simulink model "FOC_IM_discrete"  (R2018b)
settings: Solver=ode45  StartTime=0.0  StopTime=0.1  RelTol=1e-6
undefined symbols (not defined in the file): DiscIntNeverNeededParam, fs, In, J, Ki_d, Ki_q, Ki_speed, Kp_d, Kp_q, Kp_speed, landa_r, Lm, Lr, Ls, Omegae, p, plecs, Rr, Rs, T_rated, Ts, Udc, Un
libraries: powerlib_meascontrol x1, powerlib x1
settings Model: SimulationMode=accelerator  Creator=estef  LastModifiedBy=estef
settings DebuggingCC: MaxConsecutiveZCsMsg=warning

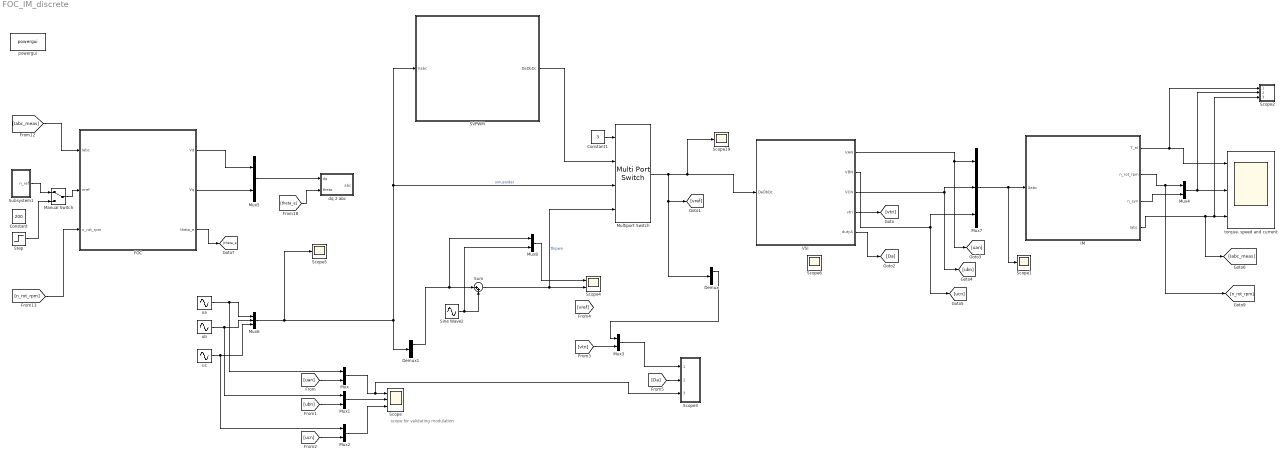
== system FOC_IM_discrete ==
  note: scope for validating modulation
  Constant : Constant  Value=200
  Constant1 : Constant  Value=3
  Demux : Demux  Outputs=3
  Demux1 : Demux  Outputs=3
  "FOC " : Subsystem
  "IM " : Subsystem
  Manual Switch : ManualSwitch
  Multiport Switch : MultiPortSwitch
  Mux{,1..5,8} (7 alike) : Mux  Inputs=2
  Mux6 : Mux  Inputs=3
  Mux7 : Mux  Inputs=3
  "SVPWM " : Subsystem
  Scope : Scope  NumInputPorts=3
  Scope{1,5..6,19} (4 alike) : Scope
  Scope2 : Subsystem  LoadFcn=plecs('sl', 300);  InitFcn=plecs('sl', 314);  StartFcn=plecs('sl', 308);  StopFcn=plecs('sl', 309);  mask{Settings=<binary blob, 1484 chars, not shown>}
      mask init:
      | plecs('sl', 315);
      settings: CopyFcn=plecs('sl', 303);  DeleteFcn=plecs('sl', 305);  UndoDeleteFcn=plecs('sl', 306);  PreSaveFcn=plecs('sl', 311);  NameChangeFcn=plecs('sl', 310);  DestroyFcn=plecs('sl', 307);  OpenFcn=plecs('sl', 302);  ErrorFcn=plerrorfcn
      mask Display: plot([0.1 0.9 0.9 0.1 0.1], [0.9 0.9 0.5 0.5 0.9])
  Scope3 : Subsystem  LoadFcn=plecs('sl', 300);  InitFcn=plecs('sl', 314);  StartFcn=plecs('sl', 308);  StopFcn=plecs('sl', 309);  mask{Settings=<binary blob, 1328 chars, not shown>}
      mask init:
      | plecs('sl', 315);
      settings: CopyFcn=plecs('sl', 303);  DeleteFcn=plecs('sl', 305);  UndoDeleteFcn=plecs('sl', 306);  PreSaveFcn=plecs('sl', 311);  NameChangeFcn=plecs('sl', 310);  DestroyFcn=plecs('sl', 307);  OpenFcn=plecs('sl', 302);  ErrorFcn=plerrorfcn
      mask Display: plot([0.1 0.9 0.9 0.1 0.1], [0.9 0.9 0.5 0.5 0.9])
  Scope4 : Scope  NumInputPorts=2
  Sine Wave2 : Sin  Amplitude=sqrt(2)*Un/5  Frequency=3*Omegae  SampleTime=0
  Step : Step  Time=0.2  After=500  SampleTime=0
  Subsystem1 : Subsystem
  Sum : Sum  Inputs=|++
  VSI : Subsystem
  dq 2 abc : Subsystem
  powergui : powerlib/powergui  Priority=1  SimulationMode=Continuous  SampleTime=50e-6  frequency=60  Iterations=50  frequencyindice=60  Pbase=100e6  ErrMax=1e-4  UnitsV=kV  UnitsW=MW  buscounter=0  FunctionMessages=off  echomessages=off  EnableUseOfTLC=off  CurrentSourceSwitches=off  DisableSnubberDevices=off  DisableRonSwitches=off  DisableVfSwitches=off  DisplayEquations=off  SolverType=Tustin/Backward Euler (TBE)  Interpol=off  ExternalGateDelay=off  methode=off  Ts=100  x0status=blocks  SPID=on  SwTol=0  HookPort=off  RestoreLinks=warning  ResistiveCurrentMeasurement=off  Frange=[0:2:500]  Ylog=off  Xlog=on  ShowGrid=off  save=off  variable=ZData  structure=phase_V  ZoomFFT=off  StartTime=0.1  cycles=10  DisplayStyle=1  fundamental=58  FreqAxis=off  MaxFrequency=1000  frequencyindicesteady=1  RmsSteady=1  display=off
  "torque, speed and current " : Scope  NumInputPorts=3
  ua : Sin  Amplitude=sqrt(2)*Un  Frequency=Omegae  SampleTime=0
  ub : Sin  Amplitude=sqrt(2)*Un  Frequency=Omegae  Phase=-2*pi/3  SampleTime=0
  uc : Sin  Amplitude=sqrt(2)*Un  Frequency=Omegae  Phase=2*pi/3  SampleTime=0
  wires:
  Mux7/1 -> Scope1/1, "IM "/1("Uabc ")
  ub/1 -> Mux1/1, Mux6/2
  [ubn] -> Mux1/2
  [ucn] -> Mux2/2
  [theta_e] -> dq 2 abc/2(theta)
  VSI/3(VCN) -> Mux7/3, [ucn]
  ua/1 -> Mux/1, Mux6/1
  [uan] -> Mux/2
  Mux1/1 -> Scope/2
  Mux5/1 -> dq 2 abc/1(dq)
  "IM "/1(T_el) -> Scope2/1(1), "torque, speed and current "/1
  uc/1 -> Mux2/1, Mux6/3
  VSI/1("VAN ") -> [uan], Mux7/1
  Mux2/1 -> Scope/3
  VSI/2("VBN ") -> Mux7/2, [ubn]
  Mux/1 -> Scope3/3(3), Scope/1
  "IM "/4(Iabc) -> [Iabc_meas], Scope2/3(3), "torque, speed and current "/3
  "FOC "/1(Vd) -> Mux5/1
  [Iabc_meas] -> "FOC "/1("Iabc ")
  "FOC "/2("Vq ") -> Mux5/2
  [n_rot_rpm] -> "FOC "/3("n_rot_rpm ")
  Manual Switch/1 -> "FOC "/2(nref)
  Subsystem1/1(n_ref) -> Manual Switch/1
  "FOC "/3("theta_e ") -> [theta_e]
  Mux4/1 -> Scope2/2(2), "torque, speed and current "/2
  "IM "/2("n_rot_rpm ") -> [n_rot_rpm], Mux4/1
  "IM "/3("n_syn ") -> Mux4/2
  Step/1 -> Manual Switch/2
  Constant1/1 -> Multiport Switch/1
  Multiport Switch/1 -> Demux/1, [vref], Scope19/1, VSI/1(DaDbDc)
  "SVPWM "/1(DaDbDc) -> Multiport Switch/2
  Mux6/1 -> Scope5/1, Multiport Switch/3, "SVPWM "/1("Vabc "), Demux1/1  "sinusoidal"
  Sine Wave2/1 -> Mux8/2, Sum/2
  Sum/1 -> Scope4/2, Multiport Switch/4  "thipwn"
  VSI/4("vtri ") -> [vtri]
  [vtri] -> Mux3/2
  Mux3/1 -> Scope3/1(1)
  VSI/5("dutyA ") -> [Da]
  [Da] -> Scope3/2(2)
  Demux/1 -> Mux3/1
  Demux1/1 -> Mux8/1, Sum/1
  Mux8/1 -> Scope4/1

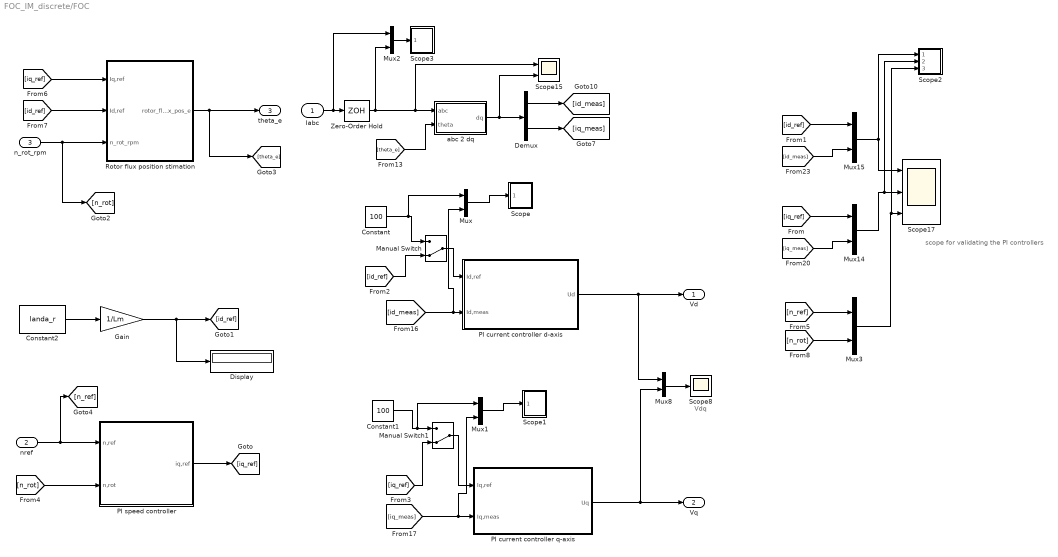
== system FOC_IM_discrete/FOC  ==
  note: scope for validating the PI controllers
  note: Vdq
  "Iabc " : Inport
  nref : Inport  Port=2
  "n_rot_rpm " : Inport  Port=3
  Constant : Constant  Value=100
  Constant1 : Constant  Value=100
  Constant2 : Constant  Value=landa_r
  Demux : Demux  Outputs=2
  Display : Display
  Gain : Gain  Gain=1/Lm
  Manual Switch : ManualSwitch  CurrentSetting=0
  Manual Switch1 : ManualSwitch  CurrentSetting=0
  Mux{,1..3,8,14..15} (7 alike) : Mux  Inputs=2
  PI current controller d-axis : Subsystem
  PI current controller q-axis : Subsystem
  PI speed controller : Subsystem
  Rotor flux position stimation : Subsystem
  Scope : Subsystem  LoadFcn=plecs('sl', 300);  InitFcn=plecs('sl', 314);  StartFcn=plecs('sl', 308);  StopFcn=plecs('sl', 309);  mask{Settings=<binary blob, 1052 chars, not shown>}
      mask init:
      | plecs('sl', 315);
      settings: CopyFcn=plecs('sl', 303);  DeleteFcn=plecs('sl', 305);  UndoDeleteFcn=plecs('sl', 306);  PreSaveFcn=plecs('sl', 311);  NameChangeFcn=plecs('sl', 310);  DestroyFcn=plecs('sl', 307);  OpenFcn=plecs('sl', 302);  ErrorFcn=plerrorfcn
      mask Display: plot([0.1 0.9 0.9 0.1 0.1], [0.9 0.9 0.5 0.5 0.9])
  Scope1 : Subsystem  LoadFcn=plecs('sl', 300);  InitFcn=plecs('sl', 314);  StartFcn=plecs('sl', 308);  StopFcn=plecs('sl', 309);  mask{Settings=<binary blob, 1052 chars, not shown>}
      mask init:
      | plecs('sl', 315);
      settings: CopyFcn=plecs('sl', 303);  DeleteFcn=plecs('sl', 305);  UndoDeleteFcn=plecs('sl', 306);  PreSaveFcn=plecs('sl', 311);  NameChangeFcn=plecs('sl', 310);  DestroyFcn=plecs('sl', 307);  OpenFcn=plecs('sl', 302);  ErrorFcn=plerrorfcn
      mask Display: plot([0.1 0.9 0.9 0.1 0.1], [0.9 0.9 0.5 0.5 0.9])
  Scope15 : Scope  NumInputPorts=2
  Scope17 : Scope  NumInputPorts=3
  Scope2 : Subsystem  LoadFcn=plecs('sl', 300);  InitFcn=plecs('sl', 314);  StartFcn=plecs('sl', 308);  StopFcn=plecs('sl', 309);  mask{Settings=<binary blob, 1952 chars, not shown>}
      mask init:
      | plecs('sl', 315);
      settings: CopyFcn=plecs('sl', 303);  DeleteFcn=plecs('sl', 305);  UndoDeleteFcn=plecs('sl', 306);  PreSaveFcn=plecs('sl', 311);  NameChangeFcn=plecs('sl', 310);  DestroyFcn=plecs('sl', 307);  OpenFcn=plecs('sl', 302);  ErrorFcn=plerrorfcn
      mask Display: plot([0.1 0.9 0.9 0.1 0.1], [0.9 0.9 0.5 0.5 0.9])
  Scope3 : Subsystem  LoadFcn=plecs('sl', 300);  InitFcn=plecs('sl', 314);  StartFcn=plecs('sl', 308);  StopFcn=plecs('sl', 309);  mask{Settings=<binary blob, 1052 chars, not shown>}
      mask init:
      | plecs('sl', 315);
      settings: CopyFcn=plecs('sl', 303);  DeleteFcn=plecs('sl', 305);  UndoDeleteFcn=plecs('sl', 306);  PreSaveFcn=plecs('sl', 311);  NameChangeFcn=plecs('sl', 310);  DestroyFcn=plecs('sl', 307);  OpenFcn=plecs('sl', 302);  ErrorFcn=plerrorfcn
      mask Display: plot([0.1 0.9 0.9 0.1 0.1], [0.9 0.9 0.5 0.5 0.9])
  Scope8 : Scope
  Zero-Order Hold : ZeroOrderHold  SampleTime=Ts
  abc 2 dq : Subsystem
  Vd : Outport
  "Vq " : Outport  Port=2
  "theta_e " : Outport  Port=3
  wires:
  Mux8/1 -> Scope8/1
  Mux15/1 -> Scope2/1(1), Scope17/1
  [id_meas] -> Mux15/2
  [iq_meas] -> Mux14/2
  Demux/2 -> [iq_meas]
  [theta_e] -> abc 2 dq/2(theta)
  abc 2 dq/1(dq) -> Scope15/2, Demux/1
  Demux/1 -> [id_meas]
  [iq_ref] -> Mux14/1
  [id_ref] -> Mux15/1
  Mux14/1 -> Scope2/2(2), Scope17/2
  PI current controller d-axis/1(Ud) -> Vd/1, Mux8/1
  [id_meas] -> Mux/2, PI current controller d-axis/2(Id,meas)
  PI current controller q-axis/1("Uq ") -> "Vq "/1, Mux8/2
  [iq_meas] -> Mux1/2, PI current controller q-axis/2(Iq,meas)
  Rotor flux position stimation/1(rotor_flux_pos_e) -> [theta_e], "theta_e "/1
  [iq_ref] -> Rotor flux position stimation/1(Iq,ref)
  [id_ref] -> Rotor flux position stimation/2(Id,ref)
  "n_rot_rpm "/1 -> [n_rot], Rotor flux position stimation/3(n_rot_rpm)
  Gain/1 -> Display/1, [id_ref]
  Constant2/1 -> Gain/1
  PI speed controller/1("iq,ref ") -> [iq_ref]
  [n_rot] -> PI speed controller/2("n,rot ")
  nref/1 -> [n_ref], PI speed controller/1(n,ref)
  [n_ref] -> Mux3/1
  [n_rot] -> Mux3/2
  Mux3/1 -> Scope2/3(3), Scope17/3
  Constant/1 -> Mux/1, Manual Switch/1
  [id_ref] -> Manual Switch/2
  Manual Switch/1 -> PI current controller d-axis/1(Id,ref)
  Constant1/1 -> Mux1/1, Manual Switch1/1
  [iq_ref] -> Manual Switch1/2
  Manual Switch1/1 -> PI current controller q-axis/1("Iq,ref ")
  Mux/1 -> Scope/1(1)
  Mux1/1 -> Scope1/1(1)
  "Iabc "/1 -> Mux2/1, Zero-Order Hold/1
  Zero-Order Hold/1 -> Scope15/1, abc 2 dq/1(abc), Mux2/2
  Mux2/1 -> Scope3/1(1)

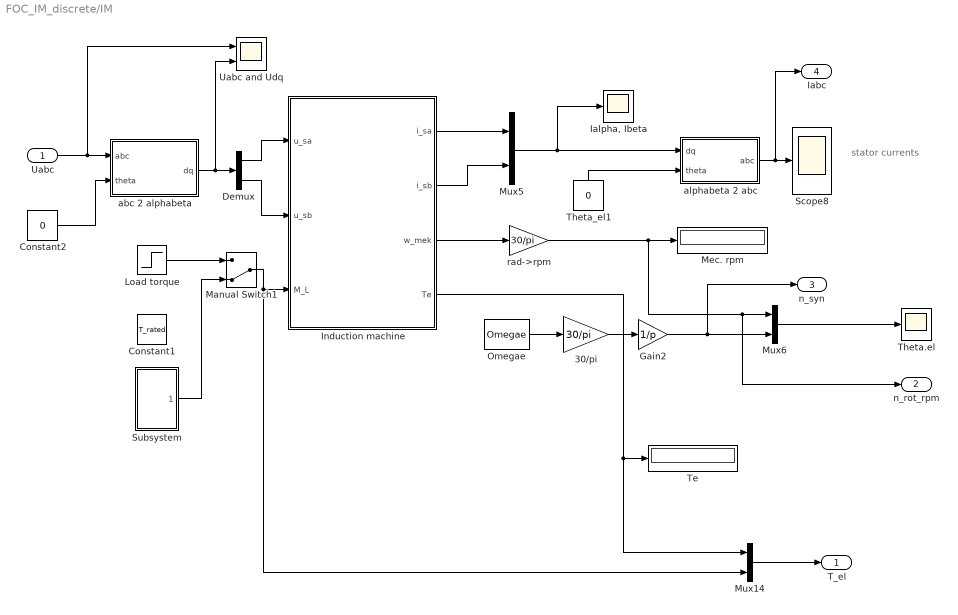
== system FOC_IM_discrete/IM  ==
  note: stator currents
  "Uabc " : Inport
  30/pi : Gain  Gain=30/pi
  Constant1 : Constant  Value=T_rated
  Constant2 : Constant  Value=0
  Demux : Demux  Outputs=2
  Gain2 : Gain  Gain=1/p
  "Ialpha, Ibeta" : Scope
  "Induction machine " : Subsystem
  Load torque : Step  After=T_rated  SampleTime=0
  Manual Switch1 : ManualSwitch  CurrentSetting=0
  Mec. rpm : Display
  Mux14 : Mux  Inputs=2
  Mux5 : Mux  Inputs=2
  Mux6 : Mux  Inputs=2
  Omegae : Constant  Value=Omegae
  Scope8 : Scope
  Subsystem : Subsystem
  Te : Display
  Theta.el : Scope
  Theta_el1 : Constant  Value=0
  Uabc and Udq : Scope  NumInputPorts=2
  abc 2 alphabeta : Subsystem
  alphabeta 2 abc : Subsystem
  rad->rpm : Gain  Gain=30/pi  SaturateOnIntegerOverflow=on  OutDataTypeStr=Inherit: Same as input  ParamDataTypeStr=Inherit: Same as input
  T_el : Outport
  "n_rot_rpm " : Outport  Port=2
  "n_syn " : Outport  Port=3
  Iabc : Outport  Port=4
  wires:
  rad->rpm/1 -> Mec. rpm/1, Mux6/1, "n_rot_rpm "/1
  "Induction machine "/4(Te) -> Mux14/1, Te/1
  Constant2/1 -> abc 2 alphabeta/2(theta)
  Manual Switch1/1 -> Mux14/2, "Induction machine "/3(M_L)
  Mux6/1 -> Theta.el/1
  abc 2 alphabeta/1(dq) -> Uabc and Udq/2, Demux/1
  Theta_el1/1 -> alphabeta 2 abc/2(theta)
  Mux14/1 -> T_el/1
  Mux5/1 -> "Ialpha, Ibeta"/1, alphabeta 2 abc/1(dq)
  "Induction machine "/1(i_sa) -> Mux5/1
  30/pi/1 -> Gain2/1
  "Induction machine "/3(w_mek) -> rad->rpm/1
  "Induction machine "/2(i_sb) -> Mux5/2
  Gain2/1 -> "n_syn "/1, Mux6/2
  Demux/1 -> "Induction machine "/1(u_sa)
  Omegae/1 -> 30/pi/1
  Demux/2 -> "Induction machine "/2(u_sb)
  "Uabc "/1 -> Uabc and Udq/1, abc 2 alphabeta/1(abc)
  Load torque/1 -> Manual Switch1/1
  alphabeta 2 abc/1(abc) -> Iabc/1, Scope8/1
  Subsystem/1(T_load) -> Manual Switch1/2

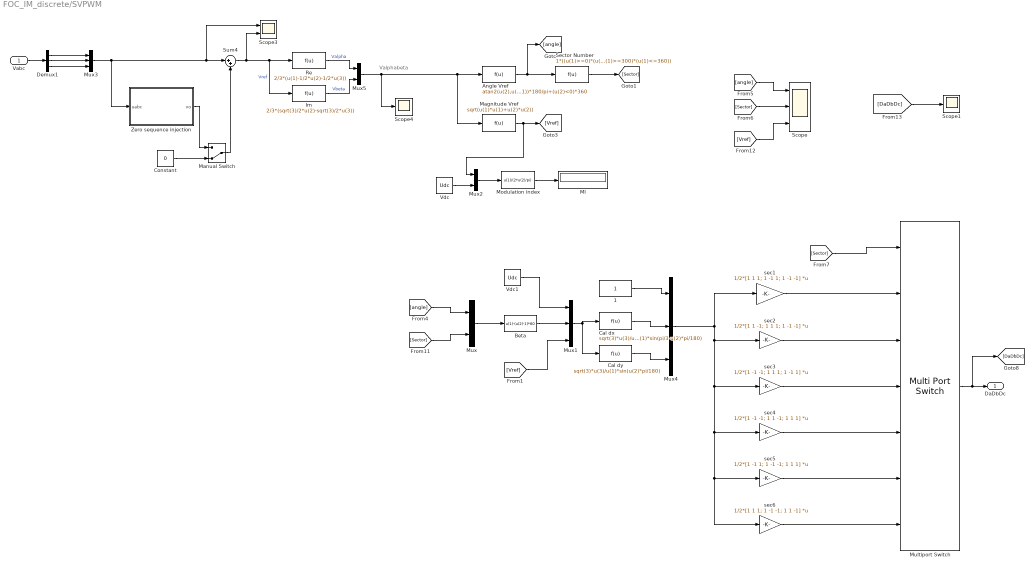
== system FOC_IM_discrete/SVPWM  ==
  note: Valphabeta
  "Vabc " : Inport
  1 : Constant
  Angle Vref : Fcn  Expr=atan2(u(2),u(1))*180/pi+(u(2)<0)*360
  Beta : Fcn  Expr=u(1)-(u(2)-1)*60
  Cal dx : Fcn  Expr=sqrt(3)*u(3)/u(1)*sin(pi/3-u(2)*pi/180)
  Cal dy : Fcn  Expr=sqrt(3)*u(3)/u(1)*sin(u(2)*pi/180)
  Constant : Constant  Value=0
  Demux1 : Demux  Outputs=3
  Im : Fcn  Expr=2/3*(sqrt(3)/2*u(2)-sqrt(3)/2*u(3))
  MI : Display
  "Magnitude Vref " : Fcn  Expr=sqrt(u(1)*u(1)+u(2)*u(2))
  Manual Switch : ManualSwitch  CurrentSetting=0
  Modulation index : Fcn  Expr=u(1)/(2*u(2)/pi)
  Multiport Switch : MultiPortSwitch  Inputs=6
  Mux : Mux  Inputs=2
  Mux1 : Mux  Inputs=3
  Mux2 : Mux  Inputs=2
  Mux3 : Mux  Inputs=3
  Mux4 : Mux  Inputs=3
  Mux5 : Mux  Inputs=2
  Re : Fcn  Expr=2/3*(u(1)-1/2*u(2)-1/2*u(3))
  Scope : Scope  NumInputPorts=3
  Scope1 : Scope
  Scope3 : Scope  NumInputPorts=2
  Scope4 : Scope
  Sector Number : Fcn  Expr=1*((u(1)>=0)*(u(1)<60))+2*((u(1)>=60)*(u(1)<120))+3*((u(1)>=120)*(u(1)<180))+4*((u(1)>=180)*(u(1)<240))+5*((u(1)>=240)*(u(1)<300))+6*((u(1)>=300)*(u(1)<=360))
  Sum4 : Sum  Inputs=|++
  Vdc : Constant  Value=Udc
  Vdc1 : Constant  Value=Udc
  Zero sequence injection : Subsystem
  sec1 : Gain  Gain=1/2*[1 1 1; 1 -1 1; 1 -1 -1]  Multiplication=Matrix(K*u)
  sec2 : Gain  Gain=1/2*[1 1 -1; 1 1 1; 1 -1 -1]  Multiplication=Matrix(K*u)
  sec3 : Gain  Gain=1/2*[1 -1 -1; 1 1 1; 1 -1 1]  Multiplication=Matrix(K*u)
  sec4 : Gain  Gain=1/2*[1 -1 -1; 1 1 -1; 1 1 1]  Multiplication=Matrix(K*u)
  sec5 : Gain  Gain=1/2*[1 -1 1; 1 -1 -1; 1 1 1]  Multiplication=Matrix(K*u)
  sec6 : Gain  Gain=1/2*[1 1 1; 1 -1 -1; 1 1 -1]  Multiplication=Matrix(K*u)
  DaDbDc : Outport
  wires:
  sec1/1 -> Multiport Switch/2
  Modulation index/1 -> MI/1
  sec3/1 -> Multiport Switch/4
  Mux2/1 -> Modulation index/1
  Mux5/1 -> "Magnitude Vref "/1, Angle Vref/1, Scope4/1
  Sector Number/1 -> [Sector]
  sec4/1 -> Multiport Switch/5
  "Magnitude Vref "/1 -> Mux2/1, [Vref]
  Angle Vref/1 -> [angle], Sector Number/1
  sec5/1 -> Multiport Switch/6
  Vdc/1 -> Mux2/2
  sec2/1 -> Multiport Switch/3
  sec6/1 -> Multiport Switch/7
  [angle] -> Scope/1
  [Sector] -> Scope/2
  [Vref] -> Scope/3
  [DaDbDc] -> Scope1/1
  Mux/1 -> Beta/1
  [angle] -> Mux/1
  [Sector] -> Mux/2
  Beta/1 -> Mux1/2
  Vdc1/1 -> Mux1/1
  [Vref] -> Mux1/3
  Mux1/1 -> Cal dx/1, Cal dy/1
  1/1 -> Mux4/1
  Cal dx/1 -> Mux4/2
  Cal dy/1 -> Mux4/3
  Mux4/1 -> sec6/1, sec5/1, sec4/1, sec3/1, sec2/1, sec1/1
  Multiport Switch/1 -> DaDbDc/1, [DaDbDc]
  [Sector] -> Multiport Switch/1
  Zero sequence injection/1("vo ") -> Manual Switch/1
  Manual Switch/1 -> Sum4/2
  Demux1/1 -> Mux3/1
  Demux1/2 -> Mux3/2
  Im/1 -> Mux5/2  "Vbeta"
  Demux1/3 -> Mux3/3
  Sum4/1 -> Scope3/2, Im/1, Re/1  "Vref"
  Constant/1 -> Manual Switch/2
  Re/1 -> Mux5/1  "Valpha"
  Mux3/1 -> Scope3/1, Sum4/1, Zero sequence injection/1(uabc)
  "Vabc "/1 -> Demux1/1

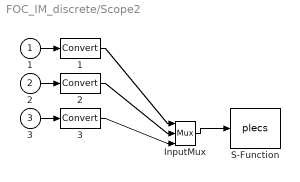
== system FOC_IM_discrete/Scope2 ==
  1 : Inport
  2 : Inport  Port=2
  3 : Inport  Port=3
  " 1 " : DataTypeConversion  SaturateOnIntegerOverflow=on  RndMeth=Zero
  " 2 " : DataTypeConversion  SaturateOnIntegerOverflow=on  RndMeth=Zero
  " 3 " : DataTypeConversion  SaturateOnIntegerOverflow=on  RndMeth=Zero
  " InputMux " : Mux  Inputs=3
  " S-Function " : S-Function  FunctionName=plecs  SFunctionDeploymentMode=off  EnableBusSupport=off
  wires:
  " InputMux "/1 -> " S-Function "/1
  1/1 -> " 1 "/1
  " 1 "/1 -> " InputMux "/1
  2/1 -> " 2 "/1
  " 2 "/1 -> " InputMux "/2
  3/1 -> " 3 "/1
  " 3 "/1 -> " InputMux "/3

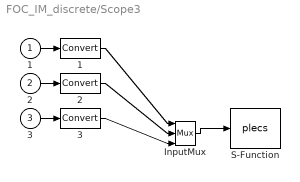
== system FOC_IM_discrete/Scope3 ==
  1 : Inport
  2 : Inport  Port=2
  3 : Inport  Port=3
  " 1 " : DataTypeConversion  SaturateOnIntegerOverflow=on  RndMeth=Zero
  " 2 " : DataTypeConversion  SaturateOnIntegerOverflow=on  RndMeth=Zero
  " 3 " : DataTypeConversion  SaturateOnIntegerOverflow=on  RndMeth=Zero
  " InputMux " : Mux  Inputs=3
  " S-Function " : S-Function  FunctionName=plecs  SFunctionDeploymentMode=off  EnableBusSupport=off
  wires:
  " InputMux "/1 -> " S-Function "/1
  1/1 -> " 1 "/1
  " 1 "/1 -> " InputMux "/1
  2/1 -> " 2 "/1
  " 2 "/1 -> " InputMux "/2
  3/1 -> " 3 "/1
  " 3 "/1 -> " InputMux "/3

== system FOC_IM_discrete/Subsystem1 ==
  Add : Sum  Inputs=+++++
  Scope4 : Scope
  Step nref 1 : Step  Time=0.3  After=500  SampleTime=0
  Step nref 2 : Step  Time=0.6  After=500  SampleTime=0
  Step nref 3 : Step  After=500  SampleTime=0
  Step nref 4 : Step  Time=1.5  After=150  SampleTime=0
  nref : Constant  Value=0.0
  n_ref : Outport
  wires:
  Add/1 -> Scope4/1, n_ref/1
  Step nref 1/1 -> Add/2
  nref/1 -> Add/1
  Step nref 2/1 -> Add/3
  Step nref 3/1 -> Add/4
  Step nref 4/1 -> Add/5

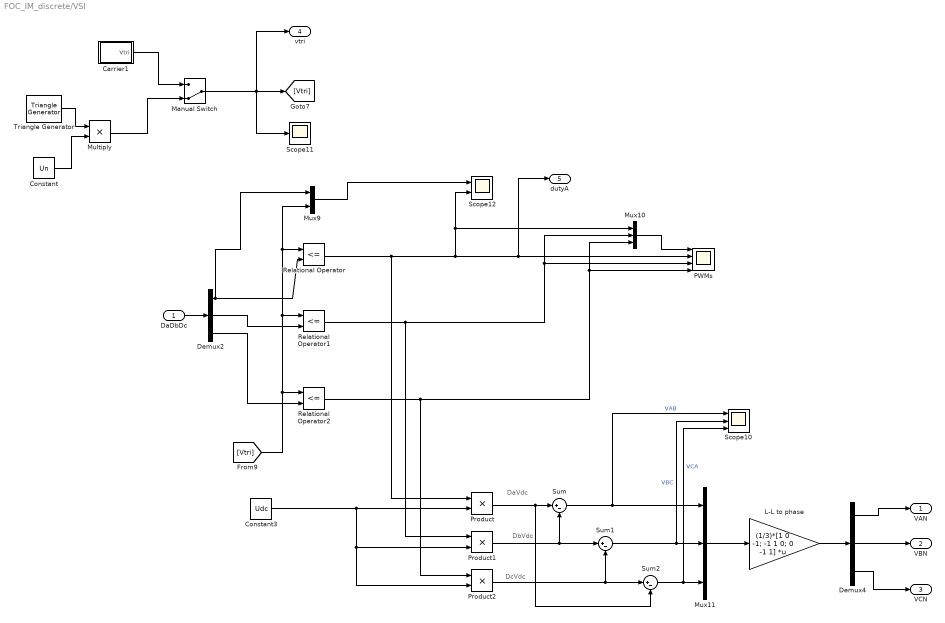
== system FOC_IM_discrete/VSI ==
  note: DcVdc
  note: DaVdc
  note: DbVdc
  DaDbDc : Inport
  Carrier1 : Subsystem  mask{fsw=fs}
      mask prompts: fsw "switching frequency"
      mask init:
      | fsw2=fsw*2;
      | x=[0 1/4 3/4 1];
      | y=[0 -1     1    0];
      mask Display: plot([x  x+1 ],[y y])
  Constant : Constant  Value=Un
  Constant3 : Constant  Value=Udc
  Demux2 : Demux  Outputs=3
  Demux4 : Demux  Outputs=3
  "L-L to phase " : Gain  Gain=(1/3)*[1 0 -1; -1 1 0; 0 -1 1]  Multiplication=Matrix(K*u)
  Manual Switch : ManualSwitch  CurrentSetting=0
  Multiply : Product
  Mux10 : Mux  Inputs=3
  Mux11 : Mux  Inputs=3
  Mux9 : Mux  Inputs=2
  "PWMs " : Scope  NumInputPorts=4
  Product : Product
  Product1 : Product
  Product2 : Product
  Relational Operator : RelationalOperator  Operator=<=  OutDataTypeStr=boolean  ZeroCross=off  RndMeth=Simplest
  Relational Operator1 : RelationalOperator  Operator=<=  OutDataTypeStr=boolean  ZeroCross=off  RndMeth=Simplest
  Relational Operator2 : RelationalOperator  Operator=<=  OutDataTypeStr=boolean  ZeroCross=off  RndMeth=Simplest
  Scope10 : Scope  NumInputPorts=3
  Scope11 : Scope
  Scope12 : Scope  NumInputPorts=2
  Sum : Sum  Inputs=|+-
  Sum1 : Sum  Inputs=|+-
  Sum2 : Sum  Inputs=|+-
  Triangle Generator : powerlib_meascontrol/Pulse & Signal Generators/Triangle Generator  Freq=fs  Phase=0  Ts=0
  "VAN " : Outport
  "VBN " : Outport  Port=2
  VCN : Outport  Port=3
  "vtri " : Outport  Port=4
  "dutyA " : Outport  Port=5
  wires:
  Sum1/1 -> Scope10/2, Mux11/2  "VBC"
  Mux10/1 -> "PWMs "/1
  Constant3/1 -> Product2/2, Product1/2, Product/2
  Demux4/3 -> VCN/1
  Demux2/2 -> Relational Operator1/2
  Demux4/2 -> "VBN "/1
  Product/1 -> Sum/1, Sum2/2
  [Vtri] -> Relational Operator1/1, Mux9/2, Relational Operator/1, Relational Operator2/1
  DaDbDc/1 -> Demux2/1
  Demux2/1 -> Mux9/1, Relational Operator/2
  Demux4/1 -> "VAN "/1
  Relational Operator/1 -> "dutyA "/1, "PWMs "/2, Mux10/1, Scope12/2, Product/1
  Mux11/1 -> "L-L to phase "/1
  Product1/1 -> Sum1/1, Sum/2
  Product2/1 -> Sum2/1, Sum1/2
  Demux2/3 -> Relational Operator2/2
  Mux9/1 -> Scope12/1
  Relational Operator2/1 -> Product2/1, "PWMs "/4, Mux10/3
  Sum/1 -> Mux11/1, Scope10/1  "VAB"
  Sum2/1 -> Scope10/3, Mux11/3  "VCA"
  "L-L to phase "/1 -> Demux4/1
  Relational Operator1/1 -> "PWMs "/3, Mux10/2, Product1/1
  Carrier1/1(Vtri) -> Manual Switch/1
  Manual Switch/1 -> "vtri "/1, Scope11/1, [Vtri]
  Triangle Generator/1 -> Multiply/1
  Constant/1 -> Multiply/2
  Multiply/1 -> Manual Switch/2

== system FOC_IM_discrete/dq 2 abc ==
  dq : Inport
  theta : Inport  Port=2
  Mux1 : Mux  Inputs=2
  Mux2 : Mux  Inputs=3
  dq2a : Fcn  Expr=(cos(u(3))*u(1)-sin(u(3))*u(2))
  dq2b : Fcn  Expr=(cos(u(3)-2*pi/3)*u(1)-sin(u(3)-2*pi/3)*u(2))
  dq2c : Fcn  Expr=(cos(u(3)+2*pi/3)*u(1)-sin(u(3)+2*pi/3)*u(2))
  abc : Outport
  wires:
  Mux2/1 -> abc/1
  dq2b/1 -> Mux2/2
  dq2a/1 -> Mux2/1
  Mux1/1 -> dq2a/1, dq2c/1, dq2b/1
  theta/1 -> Mux1/2
  dq/1 -> Mux1/1
  dq2c/1 -> Mux2/3

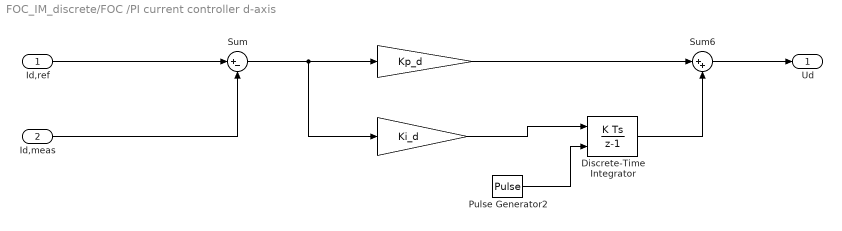
== system FOC_IM_discrete/FOC /PI current controller d-axis ==
  Id,ref : Inport
  Id,meas : Inport  Port=2
  "  " : Gain  Gain=Ki_d
  "   " : Gain  Gain=Kp_d
  Discrete-Time Integrator : DiscreteIntegrator  gainval=1  ExternalReset=rising  SampleTime=-1  UpperSaturationLimit=100  LowerSaturationLimit=-100  ICPrevOutput=DiscIntNeverNeededParam  ICPrevScaledInput=DiscIntNeverNeededParam
  Pulse Generator2 : DiscretePulseGenerator  PulseType=Time based  Period=1/fs  PulseWidth=50
  Sum : Sum  Inputs=|+-
  Sum6 : Sum  Inputs=|++
  Ud : Outport
  wires:
  Discrete-Time Integrator/1 -> Sum6/2
  "   "/1 -> Sum6/1
  Id,ref/1 -> Sum/1
  Sum/1 -> "  "/1, "   "/1
  Id,meas/1 -> Sum/2
  Sum6/1 -> Ud/1
  "  "/1 -> Discrete-Time Integrator/1
  Pulse Generator2/1 -> Discrete-Time Integrator/2

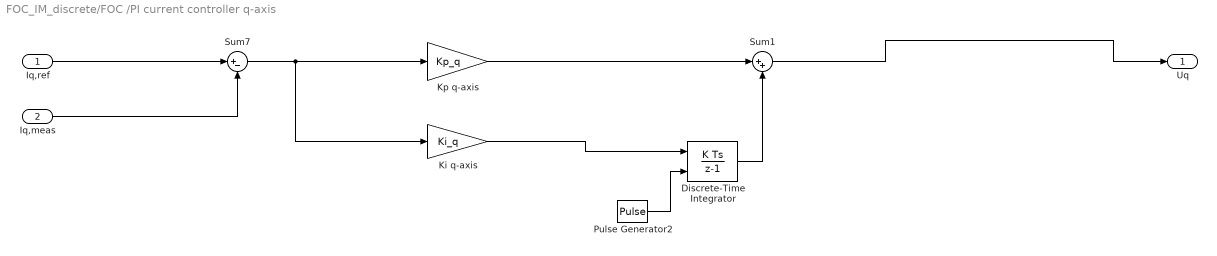
== system FOC_IM_discrete/FOC /PI current controller q-axis ==
  "Iq,ref " : Inport
  Iq,meas : Inport  Port=2
  Discrete-Time Integrator : DiscreteIntegrator  gainval=1  ExternalReset=rising  SampleTime=-1  UpperSaturationLimit=100  LowerSaturationLimit=-100  ICPrevOutput=DiscIntNeverNeededParam  ICPrevScaledInput=DiscIntNeverNeededParam
  "Ki q-axis " : Gain  Gain=Ki_q
  Kp q-axis : Gain  Gain=Kp_q
  Pulse Generator2 : DiscretePulseGenerator  PulseType=Time based  Period=1/fs  PulseWidth=50
  Sum1 : Sum  Inputs=|++
  Sum7 : Sum  Inputs=|+-  SaturateOnIntegerOverflow=on  InputSameDT=on  OutDataTypeStr=Inherit: Same as first input
  "Uq " : Outport
  wires:
  Discrete-Time Integrator/1 -> Sum1/2
  Kp q-axis/1 -> Sum1/1
  Sum7/1 -> "Ki q-axis "/1, Kp q-axis/1
  "Iq,ref "/1 -> Sum7/1
  Iq,meas/1 -> Sum7/2
  Sum1/1 -> "Uq "/1
  "Ki q-axis "/1 -> Discrete-Time Integrator/1
  Pulse Generator2/1 -> Discrete-Time Integrator/2

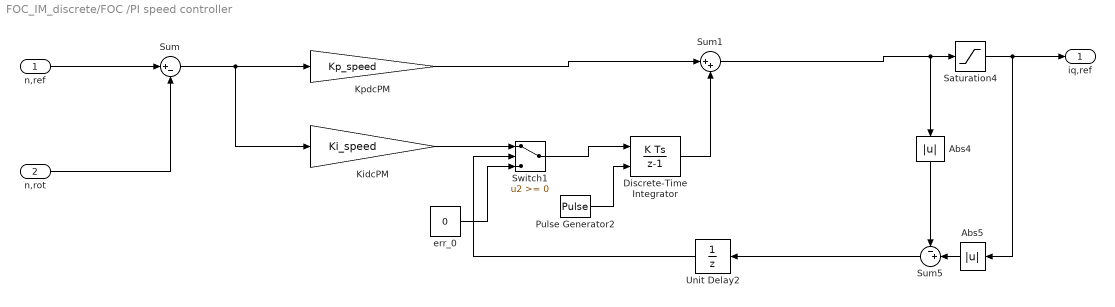
== system FOC_IM_discrete/FOC /PI speed controller ==
  n,ref : Inport
  "n,rot " : Inport  Port=2
  Abs4 : Abs
  Abs5 : Abs
  Discrete-Time Integrator : DiscreteIntegrator  gainval=1  ExternalReset=rising  SampleTime=-1  UpperSaturationLimit=100  LowerSaturationLimit=-100  ICPrevOutput=DiscIntNeverNeededParam  ICPrevScaledInput=DiscIntNeverNeededParam
  KidcPM : Gain  Gain=Ki_speed
  KpdcPM : Gain  Gain=Kp_speed
  Pulse Generator2 : DiscretePulseGenerator  PulseType=Time based  Period=1/fs  PulseWidth=50
  Saturation4 : Saturate  UpperLimit=In*sqrt(2)  LowerLimit=-In*sqrt(2)
  Sum : Sum  Inputs=|+-
  Sum1 : Sum  Inputs=|++
  Sum5 : Sum  Inputs=-+|
  Switch1 : Switch
  Unit Delay2 : UnitDelay  SampleTime=1/fs
  err_0 : Constant  Value=0
  "iq,ref " : Outport
  wires:
  Saturation4/1 -> "iq,ref "/1, Abs5/1
  Sum1/1 -> Abs4/1, Saturation4/1
  Switch1/1 -> Discrete-Time Integrator/1
  Abs5/1 -> Sum5/2
  err_0/1 -> Switch1/3
  KpdcPM/1 -> Sum1/1
  Sum5/1 -> Unit Delay2/1
  Abs4/1 -> Sum5/1
  KidcPM/1 -> Switch1/1
  Unit Delay2/1 -> Switch1/2
  n,ref/1 -> Sum/1
  "n,rot "/1 -> Sum/2
  Sum/1 -> KidcPM/1, KpdcPM/1
  Pulse Generator2/1 -> Discrete-Time Integrator/2
  Discrete-Time Integrator/1 -> Sum1/2

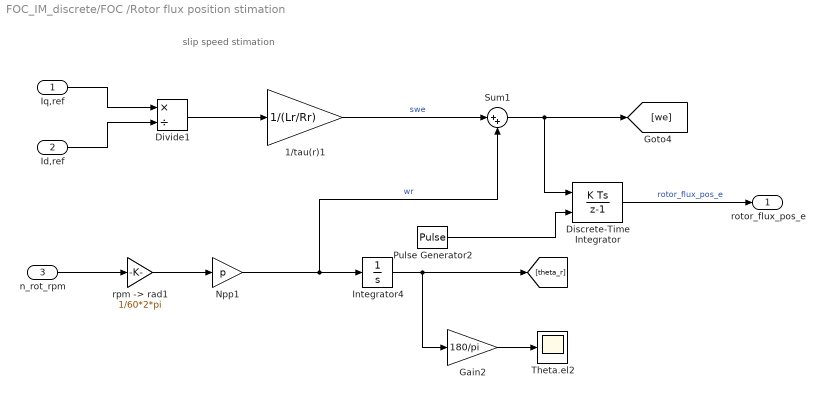
== system FOC_IM_discrete/FOC /Rotor flux position stimation ==
  note: slip speed stimation
  Iq,ref : Inport
  Id,ref : Inport  Port=2
  n_rot_rpm : Inport  Port=3
  1/tau(r)1 : Gain  Gain=1/(Lr/Rr)
  Discrete-Time Integrator : DiscreteIntegrator  gainval=1  ExternalReset=rising  SampleTime=-1  UpperSaturationLimit=100  LowerSaturationLimit=-100  ICPrevOutput=DiscIntNeverNeededParam  ICPrevScaledInput=DiscIntNeverNeededParam
  Divide1 : Product  Inputs=*/
  Gain2 : Gain  Gain=180/pi
  Integrator4 : Integrator
  Npp1 : Gain  Gain=p  SaturateOnIntegerOverflow=on  OutDataTypeStr=Inherit: Same as input  ParamDataTypeStr=Inherit: Same as input
  Pulse Generator2 : DiscretePulseGenerator  PulseType=Time based  Period=1/fs  PulseWidth=50
  Sum1 : Sum  Inputs=|++
  Theta.el2 : Scope
  "rpm -> rad1" : Gain  Gain=1/60*2*pi  SaturateOnIntegerOverflow=on  OutDataTypeStr=Inherit: Same as input  ParamDataTypeStr=Inherit: Same as input
  rotor_flux_pos_e : Outport
  wires:
  Discrete-Time Integrator/1 -> rotor_flux_pos_e/1  "rotor_flux_pos_e"
  1/tau(r)1/1 -> Sum1/1  "swe"
  Npp1/1 -> Integrator4/1, Sum1/2  "wr"
  "rpm -> rad1"/1 -> Npp1/1
  Iq,ref/1 -> Divide1/1
  Integrator4/1 -> [theta_r], Gain2/1
  Divide1/1 -> 1/tau(r)1/1
  Sum1/1 -> Discrete-Time Integrator/1, [we]
  Gain2/1 -> Theta.el2/1
  n_rot_rpm/1 -> "rpm -> rad1"/1
  Id,ref/1 -> Divide1/2
  Pulse Generator2/1 -> Discrete-Time Integrator/2

== system FOC_IM_discrete/FOC /Scope ==
  1 : Inport
  " 1 " : DataTypeConversion  SaturateOnIntegerOverflow=on  RndMeth=Zero
  " InputMux " : Mux  Inputs=1
  " S-Function " : S-Function  FunctionName=plecs  SFunctionDeploymentMode=off  EnableBusSupport=off
  wires:
  " InputMux "/1 -> " S-Function "/1
  1/1 -> " 1 "/1
  " 1 "/1 -> " InputMux "/1

== system FOC_IM_discrete/FOC /Scope1 ==
  1 : Inport
  " 1 " : DataTypeConversion  SaturateOnIntegerOverflow=on  RndMeth=Zero
  " InputMux " : Mux  Inputs=1
  " S-Function " : S-Function  FunctionName=plecs  SFunctionDeploymentMode=off  EnableBusSupport=off
  wires:
  " InputMux "/1 -> " S-Function "/1
  1/1 -> " 1 "/1
  " 1 "/1 -> " InputMux "/1

== system FOC_IM_discrete/FOC /Scope2 ==
  1 : Inport
  2 : Inport  Port=2
  3 : Inport  Port=3
  " 1 " : DataTypeConversion  SaturateOnIntegerOverflow=on  RndMeth=Zero
  " 2 " : DataTypeConversion  SaturateOnIntegerOverflow=on  RndMeth=Zero
  " 3 " : DataTypeConversion  SaturateOnIntegerOverflow=on  RndMeth=Zero
  " InputMux " : Mux  Inputs=3
  " S-Function " : S-Function  FunctionName=plecs  SFunctionDeploymentMode=off  EnableBusSupport=off
  wires:
  " InputMux "/1 -> " S-Function "/1
  1/1 -> " 1 "/1
  " 1 "/1 -> " InputMux "/1
  2/1 -> " 2 "/1
  " 2 "/1 -> " InputMux "/2
  3/1 -> " 3 "/1
  " 3 "/1 -> " InputMux "/3

== system FOC_IM_discrete/FOC /Scope3 ==
  1 : Inport
  " 1 " : DataTypeConversion  SaturateOnIntegerOverflow=on  RndMeth=Zero
  " InputMux " : Mux  Inputs=1
  " S-Function " : S-Function  FunctionName=plecs  SFunctionDeploymentMode=off  EnableBusSupport=off
  wires:
  " 1 "/1 -> " InputMux "/1
  1/1 -> " 1 "/1
  " InputMux "/1 -> " S-Function "/1

== system FOC_IM_discrete/FOC /abc 2 dq ==
  abc : Inport
  theta : Inport  Port=2
  Mux1 : Mux  Inputs=2
  Mux2 : Mux  Inputs=2
  abc2d : Fcn  Expr=2/3*(u(1)*cos(u(4))+u(2)*cos(u(4)-2*pi/3)+u(3)*cos(u(4)-4*pi/3))
  abc2q : Fcn  Expr=-2/3*(u(1)*sin(u(4))+u(2)*sin(u(4)-2*pi/3)+u(3)*sin(u(4)-4*pi/3))
  dq : Outport
  wires:
  abc/1 -> Mux1/1
  theta/1 -> Mux1/2
  Mux1/1 -> abc2d/1, abc2q/1
  abc2d/1 -> Mux2/1
  abc2q/1 -> Mux2/2
  Mux2/1 -> dq/1

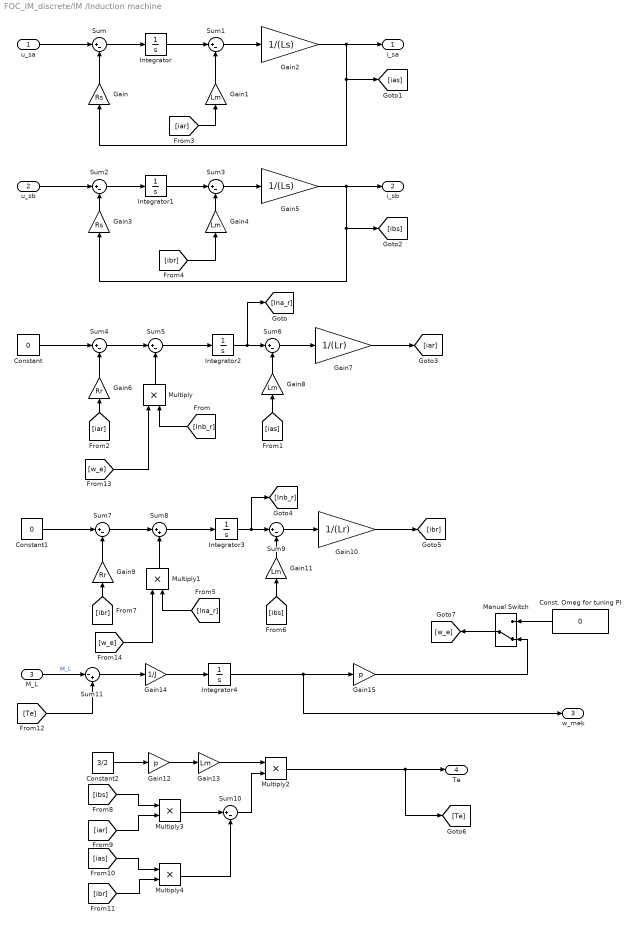
== system FOC_IM_discrete/IM /Induction machine  ==
  u_sa : Inport
  u_sb : Inport  Port=2
  M_L : Inport  Port=3
  "Const. Omeg for tuning PI " : Constant  Value=0
  Constant : Constant  Value=0
  Constant1 : Constant  Value=0
  Constant2 : Constant  Value=3/2
  Gain : Gain  Gain=Rs
  Gain{1,4,8,11,13} (5 alike) : Gain  Gain=Lm
  Gain10 : Gain  Gain=1/(Lr)
  Gain12 : Gain  Gain=p
  Gain14 : Gain  Gain=1/J
  Gain15 : Gain  Gain=p
  Gain2 : Gain  Gain=1/(Ls)
  Gain3 : Gain  Gain=Rs
  Gain5 : Gain  Gain=1/(Ls)
  Gain6 : Gain  Gain=Rr
  Gain7 : Gain  Gain=1/(Lr)
  Gain9 : Gain  Gain=Rr
  Integrator{,1..4} (5 alike) : Integrator
  Manual Switch : ManualSwitch  CurrentSetting=0
  Multiply{,1..4} (5 alike) : Product
  Sum{,1..7,9..10} (10 alike) : Sum  Inputs=|+-
  Sum11 : Sum  Inputs=|-+
  Sum8 : Sum  Inputs=|++
  i_sa : Outport
  i_sb : Outport  Port=2
  w_mek : Outport  Port=3
  Te : Outport  Port=4
  wires:
  u_sa/1 -> Sum/1
  Gain/1 -> Sum/2
  Sum/1 -> Integrator/1
  Integrator/1 -> Sum1/1
  Gain1/1 -> Sum1/2
  Sum1/1 -> Gain2/1
  Gain2/1 -> [ias], Gain/1, i_sa/1
  Gain3/1 -> Sum2/2
  u_sb/1 -> Sum2/1
  Sum3/1 -> Gain5/1
  Gain4/1 -> Sum3/2
  Gain5/1 -> i_sb/1, [ibs], Gain3/1
  Sum2/1 -> Integrator1/1
  Integrator1/1 -> Sum3/1
  Constant/1 -> Sum4/1
  Gain6/1 -> Sum4/2
  Sum4/1 -> Sum5/1
  [lnb_r] -> Multiply/2
  Sum5/1 -> Integrator2/1
  Gain8/1 -> Sum6/2
  [ias] -> Gain8/1
  Integrator2/1 -> [lna_r], Sum6/1
  Sum6/1 -> Gain7/1
  Multiply/1 -> Sum5/2
  Gain7/1 -> [iar]
  [iar] -> Gain6/1
  [ibr] -> Gain4/1
  [iar] -> Gain1/1
  Gain11/1 -> Sum9/2
  Gain10/1 -> [ibr]
  [ibr] -> Gain9/1
  [ibs] -> Gain11/1
  Multiply1/1 -> Sum8/2
  Integrator3/1 -> [lnb_r], Sum9/1
  Sum7/1 -> Sum8/1
  [lna_r] -> Multiply1/2
  Gain9/1 -> Sum7/2
  Sum9/1 -> Gain10/1
  Sum8/1 -> Integrator3/1
  Constant1/1 -> Sum7/1
  Gain13/1 -> Multiply2/1
  Sum10/1 -> Multiply2/2
  [ibs] -> Multiply3/1
  [iar] -> Multiply3/2
  Multiply3/1 -> Sum10/1
  [ias] -> Multiply4/1
  [ibr] -> Multiply4/2
  Multiply4/1 -> Sum10/2
  Constant2/1 -> Gain12/1
  Gain12/1 -> Gain13/1
  Multiply2/1 -> [Te], Te/1
  [Te] -> Sum11/2
  M_L/1 -> Sum11/1  "M_L"
  Sum11/1 -> Gain14/1
  Gain14/1 -> Integrator4/1
  [w_e] -> Multiply/1
  [w_e] -> Multiply1/1
  "Const. Omeg for tuning PI "/1 -> Manual Switch/1
  Gain15/1 -> Manual Switch/2
  Manual Switch/1 -> [w_e]
  Integrator4/1 -> w_mek/1, Gain15/1

== system FOC_IM_discrete/IM /Subsystem ==
  Add : Sum  Inputs=+++++
  Scope4 : Scope
  Step Load torque 1 : Step  Time=0.9  After=4  SampleTime=0
  Step Load torque1 : Step  Time=1.5  After=8  SampleTime=0
  Step Load torque2 : Step  Time=1.2  After=8  SampleTime=0
  Step Load torque3 : Step  Time=1.8  After=10  SampleTime=0
  Tload : Constant  Value=0.0
  T_load : Outport
  wires:
  Add/1 -> T_load/1, Scope4/1
  Step Load torque 1/1 -> Add/2
  Tload/1 -> Add/1
  Step Load torque2/1 -> Add/3
  Step Load torque1/1 -> Add/4
  Step Load torque3/1 -> Add/5

== system FOC_IM_discrete/IM /abc 2 alphabeta ==
  abc : Inport
  theta : Inport  Port=2
  Mux1 : Mux  Inputs=2
  Mux2 : Mux  Inputs=2
  abc2d : Fcn  Expr=2/3*(u(1)*cos(u(4))+u(2)*cos(u(4)-2*pi/3)+u(3)*cos(u(4)-4*pi/3))
  abc2q : Fcn  Expr=-2/3*(u(1)*sin(u(4))+u(2)*sin(u(4)-2*pi/3)+u(3)*sin(u(4)-4*pi/3))
  dq : Outport
  wires:
  abc/1 -> Mux1/1
  theta/1 -> Mux1/2
  Mux1/1 -> abc2d/1, abc2q/1
  abc2d/1 -> Mux2/1
  abc2q/1 -> Mux2/2
  Mux2/1 -> dq/1

== system FOC_IM_discrete/IM /alphabeta 2 abc ==
  dq : Inport
  theta : Inport  Port=2
  Mux1 : Mux  Inputs=2
  Mux2 : Mux  Inputs=3
  dq2a : Fcn  Expr=(cos(u(3))*u(1)-sin(u(3))*u(2))
  dq2b : Fcn  Expr=(cos(u(3)-2*pi/3)*u(1)-sin(u(3)-2*pi/3)*u(2))
  dq2c : Fcn  Expr=(cos(u(3)+2*pi/3)*u(1)-sin(u(3)+2*pi/3)*u(2))
  abc : Outport
  wires:
  Mux2/1 -> abc/1
  dq2b/1 -> Mux2/2
  dq2a/1 -> Mux2/1
  Mux1/1 -> dq2a/1, dq2c/1, dq2b/1
  theta/1 -> Mux1/2
  dq/1 -> Mux1/1
  dq2c/1 -> Mux2/3

== system FOC_IM_discrete/SVPWM /Zero sequence injection ==
  uabc : Inport
  Constant : Constant  Value=-2
  Divide : Product  Inputs=*/
  Max2 : MinMax  Function=max
  Min1 : MinMax
  Scope : Scope
  Sum7 : Sum  Inputs=|++
  "vo " : Outport
  wires:
  Sum7/1 -> Divide/1
  Constant/1 -> Divide/2
  Max2/1 -> Sum7/2
  uabc/1 -> Max2/1, Min1/1
  Divide/1 -> "vo "/1, Scope/1
  Min1/1 -> Sum7/1

== system FOC_IM_discrete/VSI/Carrier1 ==
  note: set istart time 1/fsw/4
      | set initial IC 0.5
      | to have another waveform
      |  as shown on the block
  Constant : Constant
  Constant1 : Constant  Value=2*fs
  Integrator1 : Integrator
  Product : Product  SaturateOnIntegerOverflow=on  OutDataTypeStr=Inherit: Same as first input
  Pulse Generator : DiscretePulseGenerator  PulseType=Time based  Amplitude=2  Period=1/fsw  PulseWidth=50
  Sum : Sum  Inputs=|+-  SaturateOnIntegerOverflow=on
  Vtri : Outport  InitialOutput=0
  wires:
  Pulse Generator/1 -> Sum/1
  Constant/1 -> Sum/2
  Sum/1 -> Product/1
  Constant1/1 -> Product/2
  Product/1 -> Integrator1/1
  Integrator1/1 -> Vtri/1
